simulink model "Target_Control_System"  (R2021b)
settings: Solver=FixedStepDiscrete  StartTime=0.0  StopTime=5  RelTol=1e-3
PreLoadFcn:
  | RTWConfigurationCB('preloadfcn', bdroot);
PostLoadFcn:
  | load('configuration/data_struct.mat');
  | load('configuration/fluxMaps_propMotor.mat');
  | load('configuration/parameterInit_PROP.mat');
  | load('configuration/parameterInit_PUMP.mat');
  | load('configuration/parameterInit_PITCH.mat');
  | load('configuration/parameterInit_TILT.mat');
  | %load('configuration/base_workspace_signal_definition.mat');
  | %load('resolvedatastores_to_baseworkspace_for_faster_simulation.mat');
model workspace (MAT data in the model file):
  SIMULATION_OPTIONS : Simulink.Parameter (value not decoded)
  TARGET_CODE_GEN : Simulink.Parameter (value not decoded)
  TCS_SAMPLE_FREQ_HZ : Simulink.Parameter (value not decoded)
symbols that are objects in the model workspace (value not decoded): TARGET_CODE_GEN, TCS_SAMPLE_FREQ_HZ
undefined symbols (not defined in the file): A_DQ_REF_LPF_INIT__PITCH, A_DQ_REF_LPF_INIT__PROP, A_DQ_REF_LPF_INIT__PUMP, A_DQ_REF_LPF_INIT__TILT, A_OBSERVER_CONFIDENCE_INIT__PITCH, A_OBSERVER_CONFIDENCE_INIT__PROP, A_OBSERVER_CONFIDENCE_INIT__PUMP, A_OBSERVER_CONFIDENCE_INIT__TILT, ACTUATOR_MAX_ANGLE_TRIP__PITCH, ACTUATOR_MIN_ANGLE_TRIP__PITCH, ACTUATOR_POS_SENSOR_INV_DIRECTION__PITCH, ACTUATOR_POS_SENSOR_INV_DIRECTION__TILT, ACTUATOR_POS_SENSOR_OFFSET__PITCH, ACTUATOR_POS_SENSOR_OFFSET__TILT, ADC_scaler1_baseaddr_TILT, ADC_SCALER_FLOAT_TO_FIXPOINT_EXPANSION, ANGLE_ELEC_FROM_SENSOR_OFFSET_INIT__PITCH, ANGLE_ELEC_FROM_SENSOR_OFFSET_INIT__PROP, ANGLE_ELEC_FROM_SENSOR_OFFSET_INIT__PUMP, ANGLE_ELEC_FROM_SENSOR_OFFSET_INIT__TILT, AUTO_CLEAR_FAULTS_ENABLED__PITCH, AUTO_CLEAR_FAULTS_ENABLED__PROP, AUTO_CLEAR_FAULTS_ENABLED__PUMP, AUTO_CLEAR_FAULTS_ENABLED__TILT, AUTO_CLEAR_FAULTS_WAIT_TICKS__PITCH, AUTO_CLEAR_FAULTS_WAIT_TICKS__PROP, AUTO_CLEAR_FAULTS_WAIT_TICKS__PUMP, AUTO_CLEAR_FAULTS_WAIT_TICKS__TILT, AUTO_I_ZERO_IDLE_TICKS__PITCH, AUTO_I_ZERO_IDLE_TICKS__PROP, AUTO_I_ZERO_IDLE_TICKS__PUMP, AUTO_I_ZERO_IDLE_TICKS__TILT, AUTO_I_ZERO_OFFSET_IDC_THRESHOLD__PITCH, AUTO_I_ZERO_OFFSET_IDC_THRESHOLD__PROP, AUTO_I_ZERO_OFFSET_IDC_THRESHOLD__PUMP, AUTO_I_ZERO_OFFSET_IDC_THRESHOLD__TILT, AUTO_I_ZERO_OFFSET_IPH_THRESHOLD__PITCH, AUTO_I_ZERO_OFFSET_IPH_THRESHOLD__PROP, AUTO_I_ZERO_OFFSET_IPH_THRESHOLD__PUMP, AUTO_I_ZERO_OFFSET_IPH_THRESHOLD__TILT, AUTO_SENSORLESS_SWITCHOVER_DISABLE_OMEGA, AUTO_SENSORLESS_SWITCHOVER_ENABLE_OMEGA, AUTO_SENSORLESS_SWITCHOVER_MIN_CONFIDENCE, AUXILIARY_PROTECTION_UNIT_BASEADDR__TILT, blanking_max_error_omega_INIT_PITCH, blanking_max_error_omega_INIT_TILT, blanking_max_error_position_INIT_PITCH, blanking_max_error_position_INIT_TILT, BRUTE_START_I_Q_REF_RAMP_SPEED__PITCH, BRUTE_START_I_Q_REF_RAMP_SPEED__PROP, BRUTE_START_I_Q_REF_RAMP_SPEED__PUMP, BRUTE_START_I_Q_REF_RAMP_SPEED__TILT, CONTROL_LOOP_DT_INIT__PITCH, CONTROL_LOOP_DT_INIT__PROP, CONTROL_LOOP_DT_INIT__PUMP, CONTROL_LOOP_DT_INIT__TILT, CORRECTION_FILTER_SCALE__PITCH, CORRECTION_FILTER_SCALE__PROP, CORRECTION_FILTER_SCALE__PUMP, CORRECTION_FILTER_SCALE__TILT ... (+458)
libraries: simulink x178, Reusables_Lib x24
(part 23 of 47)

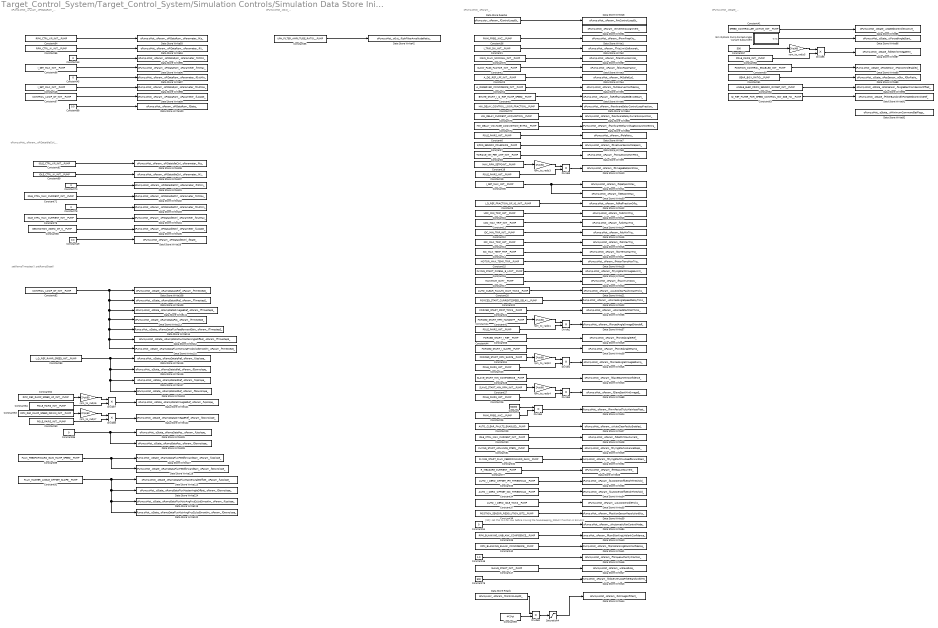
== system Target_Control_System/Target_Control_System/Simulation Controls/Simulation Data Store Initialization/parameter_init_pump/initializeMotorTaskParameterPump() ==
  note: setRampTimestep(); setRampSlope()
  note: oPump.oMot_.oParam_.oPiDataIdleCtrl_...
  note: oPump.oMot_.oParam_.oPiDataRpm_...
  note: oPump.oMot_.oState_...
  note: oPump.oMot_.oParam_...
  note: oPump.oMot_.oOut_...
  note: [SZ]: set this to 0 for now before moving the housekeeping_200Hz() function in Simulink
  Constant : Constant  Value=50000  OutDataTypeStr=single  SampleTime=-1
  Constant1 : Constant  Value=I_TRIP_SW_INIT__PUMP  OutDataTypeStr=single  SampleTime=-1
  Constant10 : Constant  Value=UDC_MIN_TRIP_INIT__PUMP  OutDataTypeStr=single  SampleTime=-1
  Constant11 : Constant  Value=UDC_MAX_TRIP_INIT__PUMP  OutDataTypeStr=single  SampleTime=-1
  Constant12 : Constant  Value=IDC_MIN_TRIP_INIT__PUMP  OutDataTypeStr=single  SampleTime=-1
  Constant13 : Constant  Value=IDC_MAX_TRIP_INIT__PUMP  OutDataTypeStr=single  SampleTime=-1
  Constant14 : Constant  Value=SIC_MAX_TEMP_TRIP__PUMP  OutDataTypeStr=single  SampleTime=-1
  Constant15 : Constant  Value=MOTOR_MAX_TEMP_TRIP__PUMP  OutDataTypeStr=single  SampleTime=-1
  Constant16 : Constant  Value=FLYING_START_OMEGA_E_LIMIT__PUMP  OutDataTypeStr=single  SampleTime=-1
  Constant17 : Constant  Value=MAXIMUM_DUTY__PUMP  OutDataTypeStr=single  SampleTime=-1
  Constant18 : Constant  Value=MAX_RPM_SETPOINT__PUMP  OutDataTypeStr=single  SampleTime=-1
  Constant{6,19,23..24,26,50,58,84} (8 alike) : Constant  Value=POLE_PAIRS_INIT__PUMP  OutDataTypeStr=single  SampleTime=-1
  Constant2 : Constant  Value=SLOW_PASS_FACTOR_INIT__PUMP  OutDataTypeStr=single  SampleTime=-1
  Constant20 : Constant  Value=AUTO_CLEAR_FAULTS_WAIT_TICKS__PUMP  OutDataTypeStr=uint32  SampleTime=-1
  Constant21 : Constant  Value=FORCED_START_POST_TICKS__PUMP  OutDataTypeStr=uint32  SampleTime=-1
  Constant22 : Constant  Value=FORCED_START_CURRENT2SPEED_DELAY__PUMP  OutDataTypeStr=uint32  SampleTime=-1
  Constant25 : Constant  Value=PWM_FREQ_KHZ__PUMP  OutDataTypeStr=single  SampleTime=-1
  Constant27 : Constant  Value=SLAVE_START_MIN_RPM_INIT__PUMP  OutDataTypeStr=single  SampleTime=-1
  Constant28 : Constant  Value=SLAVE_START_MIN_CONFIDENCE__PUMP  OutDataTypeStr=single  SampleTime=-1
  Constant29 : Constant  Value=AUTO_CLEAR_FAULTS_ENABLED__PUMP  OutDataTypeStr=uint32  SampleTime=-1
  Constant3 : Constant  Value=A_DQ_REF_LPF_INIT__PUMP  OutDataTypeStr=single  SampleTime=-1
  Constant30 : Constant  Value=IDLE_CTRL_MAX_CURRENT_INIT__PUMP  OutDataTypeStr=single  SampleTime=-1
  Constant31 : Constant  Value=FLYING_START_ADVANCE_STEPS__PUMP  OutDataTypeStr=single  SampleTime=-1
  Constant32 : Constant  Value=FLYING_START_FLUX_FEEDFORWARD_GAIN__PUMP  OutDataTypeStr=single  SampleTime=-1
  Constant33 : Constant  Value=AUTO_I_ZERO_OFFSET_IPH_THRESHOLD__PUMP  OutDataTypeStr=single  SampleTime=-1
  Constant34 : Constant  Value=AUTO_I_ZERO_OFFSET_IDC_THRESHOLD__PUMP  VectorParams1D=off  OutDataTypeStr=single  SampleTime=-1
  Constant35 : Constant  Value=I_SET_MAX_INIT__PUMP  OutDataTypeStr=single  SampleTime=-1
  Constant36 : Constant  Value=PWM_FREQ_KHZ__PUMP  OutDataTypeStr=single  SampleTime=-1
  Constant37 : Constant  Value=AUTO_I_ZERO_IDLE_TICKS__PUMP  OutDataTypeStr=uint32  SampleTime=-1
  Constant38 : Constant  Value=POSITION_SENSOR_RESOLUTION_BITS__PUMP  OutDataTypeStr=single  SampleTime=-1
  Constant39 : Constant  Value=RPM_BLANKING_UNBLANK_CONFIDENCE__PUMP  OutDataTypeStr=single  SampleTime=-1
  Constant4 : Constant  Value=A_OBSERVER_CONFIDENCE_INIT__PUMP  OutDataTypeStr=single  SampleTime=-1
  Constant40 : Constant  Value=RPM_BLANKING_BLANK_CONFIDENCE__PUMP  OutDataTypeStr=single  SampleTime=-1
  Constant41 : Constant  Value=SPEED_CONTROLLER_ACTIVE_INIT__PUMP  OutDataTypeStr=uint32  SampleTime=-1
  Constant42 : Constant  Value=FORCED_START_RPM_HANDOFF__PUMP  OutDataTypeStr=single  SampleTime=-1
  Constant{43,45,70,78,86} (5 alike) : Constant  Value=0  OutDataTypeStr=single  SampleTime=-1
  Constant44 : Constant  Value=FORCED_START_I_SLOPE__PUMP  OutDataTypeStr=single  SampleTime=-1
  Constant46 : Constant  Value=1.0  OutDataTypeStr=single  SampleTime=-1
  Constant47 : Constant  Value=SLAVE_START_INIT__PUMP  OutDataTypeStr=uint32  SampleTime=-1
  Constant48 : Constant  Value=I_SET_MAX_INIT__PUMP  OutDataTypeStr=single  SampleTime=-1
  Constant49 : Constant  Value=0.0  OutDataTypeStr=single  SampleTime=-1
  Constant5 : Constant  Value=BRUTE_START_I_Q_REF_RAMP_SPEED__PUMP  OutDataTypeStr=single  SampleTime=-1
  Constant51 : Constant  Value=FORCED_START_RPM_SLOPE__PUMP  OutDataTypeStr=single  SampleTime=-1
  Constant52 : Constant  Value=RPM_REF_RAMP_SPEED_UP_INIT__PUMP  OutDataTypeStr=single  SampleTime=-1
  Constant53 : Constant  Value=RPM_REF_RAMP_SPEED_DOWN_INIT__PUMP  OutDataTypeStr=single  SampleTime=-1
  Constant54 : Constant  Value=0  OutDataTypeStr=uint32  SampleTime=-1
  Constant55 : Constant  Value=UPH_FILTER_AMPLITUDE_RATIO__PUMP  VectorParams1D=off  OutDataTypeStr=single  SampleTime=-1
  Constant56 : Constant  Value=FORCED_START_I_REF__PUMP  OutDataTypeStr=single  SampleTime=-1
  Constant57 : Constant  Value=500  OutDataTypeStr=single  SampleTime=-1
  Constant59 : Constant  Value=4*2*pi  OutDataTypeStr=single  SampleTime=-1
  Constant60 : Constant  Value=POSITION_CONTROL_ENABLED_INIT__PUMP  OutDataTypeStr=int32  SampleTime=-1
  Constant61 : Constant  Value=GEAR_BOX_RATIO__PUMP  OutDataTypeStr=single  SampleTime=-1
  Constant62 : Constant  Value=ANGLE_ELEC_FROM_SENSOR_OFFSET_INIT__PUMP  OutDataTypeStr=single  SampleTime=-1
  Constant63 : Constant  Value=IQ_REF_FILTER_FOR_SPEED_CONTROL_BW_3DB_HZ__PUMP  OutDataTypeStr=single  SampleTime=-1
  Constant64 : Constant  Value=RPM_CTRL_KP_INIT__PUMP  OutDataTypeStr=single  SampleTime=-1
  Constant65 : Constant  Value=RPM_CTRL_KI_INIT__PUMP  OutDataTypeStr=single  SampleTime=-1
  Constant66 : Constant  Value=I_SET_MAX_INIT__PUMP  OutDataTypeStr=single  SampleTime=-1
  Constant67 : Constant  Value=CONTROL_LOOP_DT_INIT__PUMP  OutDataTypeStr=single  SampleTime=-1
  Constant68 : Constant  Value=0.0  OutDataTypeStr=single  SampleTime=-1
  Constant69 : Constant  Value=IDLE_CTRL_KI_INIT__PUMP  OutDataTypeStr=single  SampleTime=-1
  Constant7 : Constant  Value=1/POS_SENSOR_POLEPAIRS__PUMP  OutDataTypeStr=single  SampleTime=-1
  Constant71 : Constant  Value=IDLE_CTRL_MAX_CURRENT_INIT__PUMP  OutDataTypeStr=single  SampleTime=-1
  Constant72 : Constant  Value=HW_DELAY_CONTROL_LOOP_FRACTION__PUMP  OutDataTypeStr=single  SampleTime=-1
  Constant73 : Constant  Value=HW_DELAY_CURRENT_ACQUISITION__PUMP  OutDataTypeStr=single  SampleTime=-1
  Constant74 : Constant  Value=HW_DELAY_VOLTAGE_ACQUISITION_EXTRA__PUMP  OutDataTypeStr=single  SampleTime=-1
  Constant75 : Constant  Value=MAIN_FLUX_NOMINAL_INIT__PUMP  OutDataTypeStr=single  SampleTime=-1
  Constant76 : Constant  Value=500  OutDataTypeStr=single  SampleTime=-1
  Constant77 : Constant  Value=R_MEASURE_CURRENT__PUMP  OutDataTypeStr=single  SampleTime=-1
  Constant79 : Constant  Value=IDLE_CTRL_MAX_CURRENT_INIT__PUMP  VectorParams1D=off  OutDataTypeStr=single  SampleTime=-1
  Constant8 : Constant  Value=TORQUE_NM_PER_AMP_INIT__PUMP  OutDataTypeStr=single  SampleTime=-1
  Constant80 : Constant  Value=DECIMATION_200HZ_DT_S__PUMP  OutDataTypeStr=single  SampleTime=-1
  Constant81 : Constant  Value=IDLE_CTRL_KP_INIT__PUMP  OutDataTypeStr=single  SampleTime=-1
  Constant82 : Constant  Value=CONTROL_LOOP_DT_INIT__PUMP  OutDataTypeStr=single  SampleTime=-1
  Constant83 : Constant  Value=I_Q_REF_RAMP_SPEED_INIT__PUMP  OutDataTypeStr=single  SampleTime=-1
  Constant89 : Constant  Value=FLUX_FEEDFORWARD_GAIN_RAMP_SPEED__PUMP  OutDataTypeStr=single  SampleTime=-1
  Constant9 : Constant  Value=I_D_REF_FRACTION_OF_IQ_INIT__PUMP  OutDataTypeStr=single  SampleTime=-1
  Constant92 : Constant  Value=FLUX_MASTER_ANGLE_OFFSET_SLOPE__PUMP  OutDataTypeStr=single  SampleTime=-1
  Data Store Read1 : DataStoreRead  DataStoreName=oPump  DataStoreElements=oPump.oIsr_.oParam_.fControlLoopDt_  IndexOptions=Index vector (dialog)  Indices=1  OutputSizes=1
  Data Store Read14 : DataStoreRead  DataStoreName=oPump  DataStoreElements=oPump.oIsr_.oParam_.fControlLoopDt_  IndexOptions=Index vector (dialog)  Indices=1  OutputSizes=1
  Data Store Write1 : DataStoreWrite  DataStoreName=oPump  DataStoreElements=oPump.oMot_.oParam_.fPwmFreqKhz_  IndexOptions=Index vector (dialog)  Indices=1  OutputSizes=1
  Data Store Write10 : DataStoreWrite  DataStoreName=oPump  DataStoreElements=oPump.oMot_.oParam_.fOmegaESetpointMax_  IndexOptions=Index vector (dialog)  Indices=1  OutputSizes=1
  Data Store Write100 : DataStoreWrite  DataStoreName=oPump  DataStoreElements=oPump.oMot_.oParam_.oPiDataRpm_.fState_  IndexOptions=Index vector (dialog)  Indices=1  OutputSizes=1
  Data Store Write101 : DataStoreWrite  DataStoreName=oPump  DataStoreElements=oPump.oMot_.oParam_.oPiDataIdleCtrl_.oParameter_.fIntMin_  IndexOptions=Index vector (dialog)  Indices=1  OutputSizes=1
  Data Store Write102 : DataStoreWrite  DataStoreName=oPump  DataStoreElements=oPump.oMot_.oParam_.oPiDataIdleCtrl_.oParameter_.fIntMax_  IndexOptions=Index vector (dialog)  Indices=1  OutputSizes=1
  Data Store Write103 : DataStoreWrite  DataStoreName=oPump  DataStoreElements=oPump.oMot_.oParam_.oPiDataIdleCtrl_.oParameter_.fOutMin_  IndexOptions=Index vector (dialog)  Indices=1  OutputSizes=1
  Data Store Write104 : DataStoreWrite  DataStoreName=oPump  DataStoreElements=oPump.oMot_.oParam_.oPiDataIdleCtrl_.oParameter_.fOutMax_  IndexOptions=Index vector (dialog)  Indices=1  OutputSizes=1
  Data Store Write105 : DataStoreWrite  DataStoreName=oPump  DataStoreElements=oPump.oMot_.oParam_.oPiDataIdleCtrl_.oParameter_.fLoopDt_  IndexOptions=Index vector (dialog)  Indices=1  OutputSizes=1
  Data Store Write106 : DataStoreWrite  DataStoreName=oPump  DataStoreElements=oPump.oMot_.oParam_.oPiDataIdleCtrl_.oParameter_.fKp_  IndexOptions=Index vector (dialog)  Indices=1  OutputSizes=1
  Data Store Write107 : DataStoreWrite  DataStoreName=oPump  DataStoreElements=oPump.oMot_.oParam_.oPiDataIdleCtrl_.oParameter_.fKi_  IndexOptions=Index vector (dialog)  Indices=1  OutputSizes=1
  Data Store Write108 : DataStoreWrite  DataStoreName=oPump  DataStoreElements=oPump.oMot_.oState_.oRampDataIqRef_.oParam_.fTimestepS_  IndexOptions=Index vector (dialog)  Indices=1  OutputSizes=1
  Data Store Write109 : DataStoreWrite  DataStoreName=oPump  DataStoreElements=oPump.oMot_.oState_.oRampDataIdRef_.oParam_.fTimestepS_  IndexOptions=Index vector (dialog)  Indices=1  OutputSizes=1
  Data Store Write11 : DataStoreWrite  DataStoreName=oPump  DataStoreElements=oPump.oMot_.oParam_.fIqSetpointMax_  IndexOptions=Index vector (dialog)  Indices=1  OutputSizes=1
  Data Store Write110 : DataStoreWrite  DataStoreName=oPump  DataStoreElements=oPump.oMot_.oState_.oRampDataFluxMstrAngFrcd2clsdSmoothn_.oParam_.fTimestepS_  IndexOptions=Index vector (dialog)  Indices=1  OutputSizes=1
  Data Store Write111 : DataStoreWrite  DataStoreName=oPump  DataStoreElements=oPump.oMot_.oState_.oRampDataOmegaERef_.oParam_.fTimestepS_  IndexOptions=Index vector (dialog)  Indices=1  OutputSizes=1
  Data Store Write112 : DataStoreWrite  DataStoreName=oPump  DataStoreElements=oPump.oMot_.oState_.oRampDataFluxMasterAngleOffset_.oParam_.fTimestepS_  IndexOptions=Index vector (dialog)  Indices=1  OutputSizes=1
  Data Store Write113 : DataStoreWrite  DataStoreName=oPump  DataStoreElements=oPump.oMot_.oState_.oRampDataPos_.oParam_.fTimestepS_  IndexOptions=Index vector (dialog)  Indices=1  OutputSizes=1
  Data Store Write114 : DataStoreWrite  DataStoreName=oPump  DataStoreElements=oPump.oMot_.oState_.oRampDataFluxFeedforwardGain_.oParam_.fTimestepS_  IndexOptions=Index vector (dialog)  Indices=1  OutputSizes=1
  Data Store Write115 : DataStoreWrite  DataStoreName=oPump  DataStoreElements=oPump.oMot_.oState_.oRampDataIqRef_.oParam_.fUpslope_  IndexOptions=Index vector (dialog)  Indices=1  OutputSizes=1
  Data Store Write116 : DataStoreWrite  DataStoreName=oPump  DataStoreElements=oPump.oMot_.oState_.oRampDataIqRef_.oParam_.fDownslope_  IndexOptions=Index vector (dialog)  Indices=1  OutputSizes=1
  Data Store Write117 : DataStoreWrite  DataStoreName=oPump  DataStoreElements=oPump.oMot_.oState_.oRampDataIdRef_.oParam_.fUpslope_  IndexOptions=Index vector (dialog)  Indices=1  OutputSizes=1
  Data Store Write118 : DataStoreWrite  DataStoreName=oPump  DataStoreElements=oPump.oMot_.oState_.oRampDataIdRef_.oParam_.fDownslope_  IndexOptions=Index vector (dialog)  Indices=1  OutputSizes=1
  Data Store Write119 : DataStoreWrite  DataStoreName=oPump  DataStoreElements=oPump.oMot_.oState_.oRampDataFluxMstrAngFrcd2clsdSmoothn_.oParam_.fUpslope_  IndexOptions=Index vector (dialog)  Indices=1  OutputSizes=1
  Data Store Write12 : DataStoreWrite  DataStoreName=oPump  DataStoreElements=oPump.oMot_.oParam_.fIdRefFractionOfIq_  IndexOptions=Index vector (dialog)  Indices=1  OutputSizes=1
  Data Store Write120 : DataStoreWrite  DataStoreName=oPump  DataStoreElements=oPump.oMot_.oState_.oRampDataFluxMstrAngFrcd2clsdSmoothn_.oParam_.fDownslope_  IndexOptions=Index vector (dialog)  Indices=1  OutputSizes=1
  Data Store Write121 : DataStoreWrite  DataStoreName=oPump  DataStoreElements=oPump.oMot_.oState_.oRampDataOmegaERef_.oParam_.fUpslope_  IndexOptions=Index vector (dialog)  Indices=1  OutputSizes=1
  Data Store Write122 : DataStoreWrite  DataStoreName=oPump  DataStoreElements=oPump.oMot_.oState_.oRampDataOmegaERef_.oParam_.fDownslope_  IndexOptions=Index vector (dialog)  Indices=1  OutputSizes=1
  Data Store Write123 : DataStoreWrite  DataStoreName=oPump  DataStoreElements=oPump.oMot_.oState_.oRampDataFluxMasterAngleOffset_.oParam_.fUpslope_  IndexOptions=Index vector (dialog)  Indices=1  OutputSizes=1
  Data Store Write124 : DataStoreWrite  DataStoreName=oPump  DataStoreElements=oPump.oMot_.oState_.oRampDataFluxMasterAngleOffset_.oParam_.fDownslope_  IndexOptions=Index vector (dialog)  Indices=1  OutputSizes=1
  Data Store Write125 : DataStoreWrite  DataStoreName=oPump  DataStoreElements=oPump.oMot_.oState_.oRampDataPos_.oParam_.fUpslope_  IndexOptions=Index vector (dialog)  Indices=1  OutputSizes=1
  Data Store Write126 : DataStoreWrite  DataStoreName=oPump  DataStoreElements=oPump.oMot_.oState_.oRampDataPos_.oParam_.fDownslope_  IndexOptions=Index vector (dialog)  Indices=1  OutputSizes=1
  Data Store Write127 : DataStoreWrite  DataStoreName=oPump  DataStoreElements=oPump.oMot_.oState_.oRampDataFluxFeedforwardGain_.oParam_.fUpslope_  IndexOptions=Index vector (dialog)  Indices=1  OutputSizes=1
  Data Store Write128 : DataStoreWrite  DataStoreName=oPump  DataStoreElements=oPump.oMot_.oState_.oRampDataFluxFeedforwardGain_.oParam_.fDownslope_  IndexOptions=Index vector (dialog)  Indices=1  OutputSizes=1
  Data Store Write13 : DataStoreWrite  DataStoreName=oPump  DataStoreElements=oPump.oMot_.oParam_.fUdcMinTrip_  IndexOptions=Index vector (dialog)  Indices=1  OutputSizes=1
  Data Store Write14 : DataStoreWrite  DataStoreName=oPump  DataStoreElements=oPump.oMot_.oParam_.fUdcMaxTrip_  IndexOptions=Index vector (dialog)  Indices=1  OutputSizes=1
  Data Store Write15 : DataStoreWrite  DataStoreName=oPump  DataStoreElements=oPump.oMot_.oParam_.fIdcMinTrip_  IndexOptions=Index vector (dialog)  Indices=1  OutputSizes=1
  Data Store Write16 : DataStoreWrite  DataStoreName=oPump  DataStoreElements=oPump.oMot_.oParam_.fIdcMaxTrip_  IndexOptions=Index vector (dialog)  Indices=1  OutputSizes=1
  Data Store Write17 : DataStoreWrite  DataStoreName=oPump  DataStoreElements=oPump.oMot_.oParam_.fSicTempMaxTrip_  IndexOptions=Index vector (dialog)  Indices=1  OutputSizes=1
  Data Store Write18 : DataStoreWrite  DataStoreName=oPump  DataStoreElements=oPump.oMot_.oParam_.fMotorTempMaxTrip_  IndexOptions=Index vector (dialog)  Indices=1  OutputSizes=1
  Data Store Write19 : DataStoreWrite  DataStoreName=oPump  DataStoreElements=oPump.oMot_.oParam_.fFlyingStartOmegaELimit_  IndexOptions=Index vector (dialog)  Indices=1  OutputSizes=1
  Data Store Write2 : DataStoreWrite  DataStoreName=oPump  DataStoreElements=oPump.oMot_.oParam_.fTripLimitSoftwareA_  IndexOptions=Index vector (dialog)  Indices=1  OutputSizes=1
  Data Store Write20 : DataStoreWrite  DataStoreName=oPump  DataStoreElements=oPump.oMot_.oParam_.fMaximumDuty_  IndexOptions=Index vector (dialog)  Indices=1  OutputSizes=1
  Data Store Write21 : DataStoreWrite  DataStoreName=oPump  DataStoreElements=oPump.oMot_.oParam_.uiAutoClearFaultsWaitTicks_  IndexOptions=Index vector (dialog)  Indices=1  OutputSizes=1
  Data Store Write22 : DataStoreWrite  DataStoreName=oPump  DataStoreElements=oPump.oMot_.oParam_.uiForcedAngleSpeedDelayTicks_  IndexOptions=Index vector (dialog)  Indices=1  OutputSizes=1
  Data Store Write23 : DataStoreWrite  DataStoreName=oPump  DataStoreElements=oPump.oMot_.oParam_.fSlaveStartMinConfidence_  IndexOptions=Index vector (dialog)  Indices=1  OutputSizes=1
  Data Store Write24 : DataStoreWrite  DataStoreName=oPump  DataStoreElements=oPump.oMot_.oParam_.fPwmPeriodTicksMainloopFloat_  IndexOptions=Index vector (dialog)  Indices=1  OutputSizes=1
  Data Store Write25 : DataStoreWrite  DataStoreName=oPump  DataStoreElements=oPump.oMot_.oParam_.fRMeasureCurrent_  IndexOptions=Index vector (dialog)  Indices=1  OutputSizes=1
  Data Store Write26 : DataStoreWrite  DataStoreName=oPump  DataStoreElements=oPump.oMot_.oParam_.oPiDataIdleCtrl_.fState_  IndexOptions=Index vector (dialog)  Indices=1  OutputSizes=1
  Data Store Write27 : DataStoreWrite  DataStoreName=oPump  DataStoreElements=oPump.oMot_.oParam_.uiAutoClearFaultsEnabled_  IndexOptions=Index vector (dialog)  Indices=1  OutputSizes=1
  Data Store Write28 : DataStoreWrite  DataStoreName=oPump  DataStoreElements=oPump.oMot_.oParam_.fIdleCtrlMaxCurrent_  IndexOptions=Index vector (dialog)  Indices=1  OutputSizes=1
  Data Store Write29 : DataStoreWrite  DataStoreName=oPump  DataStoreElements=oPump.oMot_.oParam_.fFlyingStartAdvanceSteps_  IndexOptions=Index vector (dialog)  Indices=1  OutputSizes=1
  Data Store Write3 : DataStoreWrite  DataStoreName=oPump  DataStoreElements=oPump.oMot_.oParam_.fSlowPassFactor_  IndexOptions=Index vector (dialog)  Indices=1  OutputSizes=1
  Data Store Write30 : DataStoreWrite  DataStoreName=oPump  DataStoreElements=oPump.oMot_.oParam_.fISetpointMax_  IndexOptions=Index vector (dialog)  Indices=1  OutputSizes=1
  Data Store Write31 : DataStoreWrite  DataStoreName=oPump  DataStoreElements=oPump.oMot_.oParam_.eInverterAssignment_  IndexOptions=Index vector (dialog)  Indices=1  OutputSizes=1
  Data Store Write32 : DataStoreWrite  DataStoreName=oPump  DataStoreElements=oPump.oMot_.oParam_.fFlyingStartFluxFeedforwardGain_  IndexOptions=Index vector (dialog)  Indices=1  OutputSizes=1
  Data Store Write33 : DataStoreWrite  DataStoreName=oPump  DataStoreElements=oPump.oMot_.oParam_.fAutoIZeroOffsetIphThreshold_  IndexOptions=Index vector (dialog)  Indices=1  OutputSizes=1
  Data Store Write34 : DataStoreWrite  DataStoreName=oPump  DataStoreElements=oPump.oMot_.oParam_.fAutoIZeroOffsetIdcThreshold_  IndexOptions=Index vector (dialog)  Indices=1  OutputSizes=1
  Data Store Write35 : DataStoreWrite  DataStoreName=oPump  DataStoreElements=oPump.oMot_.oParam_.uiAutoIZeroIdleTicks_  IndexOptions=Index vector (dialog)  Indices=1  OutputSizes=1
  Data Store Write36 : DataStoreWrite  DataStoreName=oPump  DataStoreElements=oPump.oMot_.oParam_.uiForcedStartPostTicks_  IndexOptions=Index vector (dialog)  Indices=1  OutputSizes=1
  Data Store Write37 : DataStoreWrite  DataStoreName=oPump  DataStoreElements=oPump.oMot_.oParam_.fForcedAngleOmegaEHandoff_  IndexOptions=Index vector (dialog)  Indices=1  OutputSizes=1
  Data Store Write38 : DataStoreWrite  DataStoreName=oPump  DataStoreElements=oPump.oMot_.oParam_.fForcedAngleIRamp_  IndexOptions=Index vector (dialog)  Indices=1  OutputSizes=1
  Data Store Write39 : DataStoreWrite  DataStoreName=oPump  DataStoreElements=oPump.oMot_.oParam_.fPositionSensorResolutionBits_  IndexOptions=Index vector (dialog)  Indices=1  OutputSizes=1
  Data Store Write4 : DataStoreWrite  DataStoreName=oPump  DataStoreElements=oPump.oMot_.oParam_.fADqRefLpf_  IndexOptions=Index vector (dialog)  Indices=1  OutputSizes=1
  Data Store Write40 : DataStoreWrite  DataStoreName=oPump  DataStoreElements=oPump.oMot_.oParam_.fRpmBlankingUnblankConfidence_  IndexOptions=Index vector (dialog)  Indices=1  OutputSizes=1
  Data Store Write41 : DataStoreWrite  DataStoreName=oPump  DataStoreElements=oPump.oMot_.oParam_.fRpmBlankingBlankConfidence_  IndexOptions=Index vector (dialog)  Indices=1  OutputSizes=1
  Data Store Write42 : DataStoreWrite  DataStoreName=oPump  DataStoreElements=oPump.oMot_.oOut_.fUphFilterAmplitudeRatio_  IndexOptions=Index vector (dialog)  Indices=1  OutputSizes=1
  Data Store Write43 : DataStoreWrite  DataStoreName=oPump  DataStoreElements=oPump.oMot_.oParam_.fObserverLoopFilterBandwidthHz_  IndexOptions=Index vector (dialog)  Indices=1  OutputSizes=1
  Data Store Write44 : DataStoreWrite  DataStoreName=oPump  DataStoreElements=oPump.oMot_.oParam_.fAOmegaXfilter2_  IndexOptions=Index vector (dialog)  Indices=1  OutputSizes=1
  Data Store Write45 : DataStoreWrite  DataStoreName=oPump  DataStoreElements=oPump.oMot_.oParam_.fForcedAngleOmegaERamp_  IndexOptions=Index vector (dialog)  Indices=1  OutputSizes=1
  Data Store Write46 : DataStoreWrite  DataStoreName=oPump  DataStoreElements=oPump.oMot_.oParam_.fTorqueAuthorityFraction_  IndexOptions=Index vector (dialog)  Indices=1  OutputSizes=1
  Data Store Write47 : DataStoreWrite  DataStoreName=oPump  DataStoreElements=oPump.oMot_.oParam_.uiSlaveRole_  IndexOptions=Index vector (dialog)  Indices=1  OutputSizes=1
  Data Store Write48 : DataStoreWrite  DataStoreName=oPump  DataStoreElements=oPump.oMot_.oParam_.fIntControlLoopDt_  IndexOptions=Index vector (dialog)  Indices=1  OutputSizes=1
  Data Store Write49 : DataStoreWrite  DataStoreName=oPump  DataStoreElements=oPump.oMot_.oParam_.fForcedAngleIRef_  IndexOptions=Index vector (dialog)  Indices=1  OutputSizes=1
  Data Store Write5 : DataStoreWrite  DataStoreName=oPump  DataStoreElements=oPump.oMot_.oParam_.fAObserverConfidence_  IndexOptions=Index vector (dialog)  Indices=1  OutputSizes=1
  Data Store Write6 : DataStoreWrite  DataStoreName=oPump  DataStoreElements=oPump.oMot_.oParam_.fIqRefRampSpeedBruteStart_  IndexOptions=Index vector (dialog)  Indices=1  OutputSizes=1
  Data Store Write64 : DataStoreWrite  DataStoreName=oPump  DataStoreElements=oPump.oMot_.oParam_.fHardwareDelayControlLoopFraction_  IndexOptions=Index vector (dialog)  Indices=1  OutputSizes=1
  Data Store Write65 : DataStoreWrite  DataStoreName=oPump  DataStoreElements=oPump.oMot_.oParam_.fHardwareDelayCurrentAcquisition_  IndexOptions=Index vector (dialog)  Indices=1  OutputSizes=1
  Data Store Write66 : DataStoreWrite  DataStoreName=oPump  DataStoreElements=oPump.oMot_.oParam_.fHardwareDelayVoltageAcquisitionExtra_  IndexOptions=Index vector (dialog)  Indices=1  OutputSizes=1
  Data Store Write67 : DataStoreWrite  DataStoreName=oPump  DataStoreElements=oPump.oMot_.oParam_.fMainFluxNominal_  IndexOptions=Index vector (dialog)  Indices=1  OutputSizes=1
  Data Store Write69 : DataStoreWrite  DataStoreName=oPump  DataStoreElements=oPump.oMot_.oParam_.fSlaveStartMinOmegaE_  IndexOptions=Index vector (dialog)  Indices=1  OutputSizes=1
  Data Store Write7 : DataStoreWrite  DataStoreName=oPump  DataStoreElements=oPump.oMot_.oParam_.fPolePairs_  IndexOptions=Index vector (dialog)  Indices=1  OutputSizes=1
  Data Store Write8 : DataStoreWrite  DataStoreName=oPump  DataStoreElements=oPump.oMot_.oParam_.fOneOverSensorPolepairs_  IndexOptions=Index vector (dialog)  Indices=1  OutputSizes=1
  Data Store Write84 : DataStoreWrite  DataStoreName=oPump  DataStoreElements=oPump.oMot_.oParam_.uiAutomaticFanControlMode_  IndexOptions=Index vector (dialog)  Indices=1  OutputSizes=1
  Data Store Write85 : DataStoreWrite  DataStoreName=oPump  DataStoreElements=oPump.oMot_.oState_.uiSpeedControllerActive_  IndexOptions=Index vector (dialog)  Indices=1  OutputSizes=1
  Data Store Write86 : DataStoreWrite  DataStoreName=oPump  DataStoreElements=oPump.oMot_.oState_.uiForcedAngleStart_  IndexOptions=Index vector (dialog)  Indices=1  OutputSizes=1
  Data Store Write87 : DataStoreWrite  DataStoreName=oPump  DataStoreElements=oPump.oMot_.oState_.fIdleCtrlOmegaEMin_  IndexOptions=Index vector (dialog)  Indices=1  OutputSizes=1
  Data Store Write88 : DataStoreWrite  DataStoreName=oPump  DataStoreElements=oPump.oMot_.oState_.oPosSensor_.iPosControlEnabled_  IndexOptions=Index vector (dialog)  Indices=1  OutputSizes=1
  Data Store Write89 : DataStoreWrite  DataStoreName=oPump  DataStoreElements=oPump.oMot_.oState_.oPosSensor_.oGbx_.fGbxRatio_  IndexOptions=Index vector (dialog)  Indices=1  OutputSizes=1
  Data Store Write9 : DataStoreWrite  DataStoreName=oPump  DataStoreElements=oPump.oMot_.oParam_.fTorqueConstNmPerA_  IndexOptions=Index vector (dialog)  Indices=1  OutputSizes=1
  Data Store Write90 : DataStoreWrite  DataStoreName=oPump  DataStoreElements=oPump.oMot_.oState_.oPosSensor_.fAngleElecFromSensorOffset_  IndexOptions=Index vector (dialog)  Indices=1  OutputSizes=1
  Data Store Write91 : DataStoreWrite  DataStoreName=oPump  DataStoreElements=oPump.oMot_.oState_.fFilterBandwidthForSpeedControlIqRef_  IndexOptions=Index vector (dialog)  Indices=1  OutputSizes=1
  Data Store Write92 : DataStoreWrite  DataStoreName=oPump  DataStoreElements=oPump.oMot_.oState_.uiMinimumCommandSetFlags_  IndexOptions=Index vector (dialog)  Indices=1  OutputSizes=1
  Data Store Write93 : DataStoreWrite  DataStoreName=oPump  DataStoreElements=oPump.oMot_.oParam_.oPiDataRpm_.oParameter_.fKp_  IndexOptions=Index vector (dialog)  Indices=1  OutputSizes=1
  Data Store Write94 : DataStoreWrite  DataStoreName=oPump  DataStoreElements=oPump.oMot_.oParam_.oPiDataRpm_.oParameter_.fKi_  IndexOptions=Index vector (dialog)  Indices=1  OutputSizes=1
  Data Store Write95 : DataStoreWrite  DataStoreName=oPump  DataStoreElements=oPump.oMot_.oParam_.oPiDataRpm_.oParameter_.fIntMin_  IndexOptions=Index vector (dialog)  Indices=1  OutputSizes=1
  Data Store Write96 : DataStoreWrite  DataStoreName=oPump  DataStoreElements=oPump.oMot_.oParam_.oPiDataRpm_.oParameter_.fIntMax_  IndexOptions=Index vector (dialog)  Indices=1  OutputSizes=1
  Data Store Write97 : DataStoreWrite  DataStoreName=oPump  DataStoreElements=oPump.oMot_.oParam_.oPiDataRpm_.oParameter_.fOutMin_  IndexOptions=Index vector (dialog)  Indices=1  OutputSizes=1
  Data Store Write98 : DataStoreWrite  DataStoreName=oPump  DataStoreElements=oPump.oMot_.oParam_.oPiDataRpm_.oParameter_.fOutMax_  IndexOptions=Index vector (dialog)  Indices=1  OutputSizes=1
  Data Store Write99 : DataStoreWrite  DataStoreName=oPump  DataStoreElements=oPump.oMot_.oParam_.oPiDataRpm_.oParameter_.fLoopDt_  IndexOptions=Index vector (dialog)  Indices=1  OutputSizes=1
  Divide{1..8} (8 alike) : Product  Inputs=**  OutDataTypeStr=single
  Divide9 : Product  Inputs=**
  Saturation4 : Saturate  UpperLimit=1.0  LowerLimit=1e-6
  Sim Options Pump Forced Angle Variant Subsystem : Subsystem  Variant=on
  rpm_to_rad/s{1..7} (7 alike) : Gain  Gain=2*pi/60  OutDataTypeStr=single
  wires:
  Saturation4/1 -> Data Store Write44/1
  Divide9/1 -> Saturation4/1
  Constant59/1 -> Divide9/2
  Data Store Read1/1 -> Divide9/1
  Data Store Read14/1 -> Data Store Write48/1
  Constant76/1 -> Data Store Write43/1
  Constant55/1 -> Data Store Write42/1
  Constant53/1 -> rpm_to_rad/s7/1
  Constant52/1 -> rpm_to_rad/s6/1
  Divide8/1 -> Data Store Write122/1
  rpm_to_rad/s7/1 -> Divide8/1
  Constant50/1 -> Divide8/2
  Constant49/1 -> Data Store Write26/1
  Constant48/1 -> Data Store Write98/1
  Constant45/1 -> Data Store Write97/1
  Constant43/1 -> Data Store Write95/1
  Constant79/1 -> Data Store Write104/1
  Constant92/1 -> Data Store Write123/1, Data Store Write120/1, Data Store Write119/1, Data Store Write124/1
  Constant64/1 -> Data Store Write93/1
  Constant80/1 -> Data Store Write105/1
  Constant89/1 -> Data Store Write127/1, Data Store Write128/1
  Constant86/1 -> Data Store Write125/1, Data Store Write126/1
  Constant69/1 -> Data Store Write107/1
  Constant81/1 -> Data Store Write106/1
  Constant83/1 -> Data Store Write115/1, Data Store Write118/1, Data Store Write117/1, Data Store Write116/1
  Constant70/1 -> Data Store Write101/1
  rpm_to_rad/s6/1 -> Divide7/1
  Constant71/1 -> Data Store Write102/1
  Constant67/1 -> Data Store Write99/1
  Constant84/1 -> Divide7/2
  Constant78/1 -> Data Store Write103/1
  Constant66/1 -> Data Store Write96/1
  Divide7/1 -> Data Store Write121/1
  Constant68/1 -> Data Store Write100/1
  Constant65/1 -> Data Store Write94/1
  Constant82/1 -> Data Store Write110/1, Data Store Write112/1, Data Store Write114/1, Data Store Write113/1, Data Store Write111/1, Data Store Write109/1, Data Store Write108/1
  Constant57/1 -> rpm_to_rad/s5/1
  rpm_to_rad/s5/1 -> Divide6/1
  Constant63/1 -> Data Store Write91/1
  Constant41/1 -> Data Store Write85/1
  Constant61/1 -> Data Store Write89/1
  Constant58/1 -> Divide6/2
  Constant60/1 -> Data Store Write88/1
  Sim Options Pump Forced Angle Variant Subsystem/1(Out1) -> Data Store Write86/1
  Divide6/1 -> Data Store Write87/1
  Constant62/1 -> Data Store Write90/1
  Constant54/1 -> Data Store Write84/1
  Constant46/1 -> Data Store Write46/1
  Constant13/1 -> Data Store Write16/1
  Constant5/1 -> Data Store Write6/1
  Constant24/1 -> Divide2/2
  Constant33/1 -> Data Store Write33/1
  Constant31/1 -> Data Store Write29/1
  Constant16/1 -> Data Store Write19/1
  Constant18/1 -> rpm_to_rad/s3/1
  Constant37/1 -> Data Store Write35/1
  Constant40/1 -> Data Store Write41/1
  Divide5/1 -> Data Store Write69/1
  rpm_to_rad/s3/1 -> Divide3/1
  Constant47/1 -> Data Store Write47/1
  Constant2/1 -> Data Store Write3/1
  Constant11/1 -> Data Store Write14/1
  Constant36/1 -> Data Store Write1/1
  Constant14/1 -> Data Store Write17/1
  Constant75/1 -> Data Store Write67/1
  Constant30/1 -> Data Store Write28/1
  Constant74/1 -> Data Store Write66/1
  Constant26/1 -> Divide5/2
  Constant15/1 -> Data Store Write18/1
  Divide4/1 -> Data Store Write24/1
  Constant10/1 -> Data Store Write13/1
  Constant21/1 -> Data Store Write36/1
  rpm_to_rad/s2/1 -> Divide1/1
  Constant44/1 -> Data Store Write38/1
  Constant28/1 -> Data Store Write23/1
  Divide3/1 -> Data Store Write10/1
  Constant1/1 -> Data Store Write2/1
  Constant32/1 -> Data Store Write32/1
  Constant9/1 -> Data Store Write12/1
  Constant7/1 -> Data Store Write8/1
  Constant25/1 -> Divide4/2
  Constant4/1 -> Data Store Write5/1
  rpm_to_rad/s4/1 -> Divide5/1
  Constant22/1 -> Data Store Write22/1
  Constant6/1 -> Data Store Write7/1
  Divide2/1 -> Data Store Write37/1
  Constant56/1 -> Data Store Write49/1
  Constant12/1 -> Data Store Write15/1
  rpm_to_rad/s1/1 -> Divide2/1
  Constant77/1 -> Data Store Write25/1
  Constant3/1 -> Data Store Write4/1
  Constant39/1 -> Data Store Write40/1
  Constant27/1 -> rpm_to_rad/s4/1
  Constant29/1 -> Data Store Write27/1
  Constant42/1 -> rpm_to_rad/s1/1
  Constant73/1 -> Data Store Write65/1
  Constant17/1 -> Data Store Write20/1
  Constant20/1 -> Data Store Write21/1
  Constant8/1 -> Data Store Write9/1
  Constant35/1 -> Data Store Write30/1, Data Store Write11/1
  Constant/1 -> Divide4/1
  Divide1/1 -> Data Store Write45/1
  Constant19/1 -> Divide3/2
  Constant38/1 -> Data Store Write39/1
  Constant23/1 -> Divide1/2
  Constant72/1 -> Data Store Write64/1
  Constant51/1 -> rpm_to_rad/s2/1
  Constant34/1 -> Data Store Write34/1

== system Target_Control_System/Target_Control_System/Simulation Controls/Simulation Data Store Initialization/setPositionControlModeTilt()/Enabled Subsystem ==
  note: // Valid for VP and tilt, use updateIqSetpointMax(blah) for prop though;
  Enable : EnablePort
  Constant : Constant  Value=0  OutDataTypeStr=uint32  SampleTime=-1
  Constant1 : Constant  Value=I_SET_MAX_INIT__TILT_TIP  OutDataTypeStr=single  SampleTime=-1
  Constant2 : Constant  Value=I_SET_MAX_INIT__TILT_LINKAGE  OutDataTypeStr=single  SampleTime=-1
  Constant3 : Constant  OutDataTypeStr=int32  SampleTime=-1
  Constant4 : Constant  OutDataTypeStr=uint32  SampleTime=-1
  Constant5 : Constant  Value=0  OutDataTypeStr=uint32  SampleTime=-1
  Constant6 : Constant  Value=0  OutDataTypeStr=uint32  SampleTime=-1
  Constant7 : Constant  Value=0  OutDataTypeStr=single  SampleTime=-1
  Constant8 : Constant  Value=0  OutDataTypeStr=single  SampleTime=-1
  Constant9 : Constant  Value=0  OutDataTypeStr=single  SampleTime=-1
  Data Store Read : DataStoreRead  DataStoreName=oTilt  DataStoreElements=oTilt.oMot_.oState_.oPosSensor_.iTiltReadheadCompensationEnabled_  IndexOptions=Index vector (dialog)  Indices=1  OutputSizes=1
  Data Store Read1 : DataStoreRead  Commented=on  DataStoreName=oTilt  DataStoreElements=oTilt.oMot_.oParam_.ePositionControlMode_  IndexOptions=Index vector (dialog)  Indices=1  OutputSizes=1
  Data Store Read{2..8} (7 alike) : DataStoreRead  DataStoreName=oTilt  DataStoreElements=oTilt.oMot_.oParam_.fIqSetpointMax_  IndexOptions=Index vector (dialog)  Indices=1  OutputSizes=1
  Data Store Write : DataStoreWrite  DataStoreName=oTilt  DataStoreElements=oTilt.oMot_.oParam_.uiTorqueMirroringActive_  IndexOptions=Index vector (dialog)  Indices=1  OutputSizes=1
  Data Store Write1 : DataStoreWrite  DataStoreName=oTilt  DataStoreElements=oTilt.oMot_.oParam_.fISetpointMax_  IndexOptions=Index vector (dialog)  Indices=1  OutputSizes=1
  Data Store Write10 : DataStoreWrite  DataStoreName=oTilt  DataStoreElements=oTilt.oMot_.oParam_.oPid2DataRpmCtrl_.oParameter_.fDMax_  IndexOptions=Index vector (dialog)  Indices=1  OutputSizes=1
  Data Store Write11 : DataStoreWrite  DataStoreName=oTilt  DataStoreElements=oTilt.oMot_.oParam_.oPid2DataRpmCtrl_.oParameter_.fOutMin_  IndexOptions=Index vector (dialog)  Indices=1  OutputSizes=1
  Data Store Write12 : DataStoreWrite  DataStoreName=oTilt  DataStoreElements=oTilt.oMot_.oParam_.oPid2DataRpmCtrl_.oParameter_.fOutMax_  IndexOptions=Index vector (dialog)  Indices=1  OutputSizes=1
  Data Store Write13 : DataStoreWrite  Commented=on  DataStoreName=oTilt  DataStoreElements=oTilt.oMot_.oParam_.ePositionControlMode_  IndexOptions=Index vector (dialog)  Indices=1  OutputSizes=1
  Data Store Write14 : DataStoreWrite  DataStoreName=oTilt  DataStoreElements=oTilt.oMot_.oParam_.oPid2DataRpmCtrl_.oParameter_.fIntegratorLeakFactor_  IndexOptions=Index vector (dialog)  Indices=1  OutputSizes=1
  Data Store Write15 : DataStoreWrite  DataStoreName=oTilt  DataStoreElements=oTilt.oMot_.oParam_.oPid2DataRpmCtrl_.oParameter_.fErrorReduction_  IndexOptions=Index vector (dialog)  Indices=1  OutputSizes=1
  Data Store Write16 : DataStoreWrite  DataStoreName=oTilt  DataStoreElements=oTilt.oMot_.oState_.oPosSensor_.oPidDataPosCtrl_.oParameter_.fErrorReduction_  IndexOptions=Index vector (dialog)  Indices=1  OutputSizes=1
  Data Store Write2 : DataStoreWrite  DataStoreName=oTilt  DataStoreElements=oTilt.oMot_.oState_.oPosSensor_.iPosControlEnabled_  IndexOptions=Index vector (dialog)  Indices=1  OutputSizes=1
  Data Store Write3 : DataStoreWrite  DataStoreName=oTilt  DataStoreElements=oTilt.oMot_.oState_.uiSpeedControllerActive_  IndexOptions=Index vector (dialog)  Indices=1  OutputSizes=1
  Data Store Write4 : DataStoreWrite  DataStoreName=oTilt  DataStoreElements=oTilt.oMot_.oOut_.uiForcedAngle_  IndexOptions=Index vector (dialog)  Indices=1  OutputSizes=1
  Data Store Write5 : DataStoreWrite  DataStoreName=oTilt  DataStoreElements=oTilt.oMot_.oParam_.iForcedPositionHoldMode_  IndexOptions=Index vector (dialog)  Indices=1  OutputSizes=1
  Data Store Write6 : DataStoreWrite  DataStoreName=oTilt  DataStoreElements=oTilt.oMot_.oParam_.fIqSetpointMax_  IndexOptions=Index vector (dialog)  Indices=1  OutputSizes=1
  Data Store Write7 : DataStoreWrite  DataStoreName=oTilt  DataStoreElements=oTilt.oMot_.oParam_.oPid2DataRpmCtrl_.oParameter_.fIntMin_  IndexOptions=Index vector (dialog)  Indices=1  OutputSizes=1
  Data Store Write8 : DataStoreWrite  DataStoreName=oTilt  DataStoreElements=oTilt.oMot_.oParam_.oPid2DataRpmCtrl_.oParameter_.fIntMax_  IndexOptions=Index vector (dialog)  Indices=1  OutputSizes=1
  Data Store Write9 : DataStoreWrite  DataStoreName=oTilt  DataStoreElements=oTilt.oMot_.oParam_.oPid2DataRpmCtrl_.oParameter_.fDMin_  IndexOptions=Index vector (dialog)  Indices=1  OutputSizes=1
  Enumerated Constant : simulink/Sources/Enumerated Constant  Commented=on  OutDataTypeStr=Enum: EPositionControlModes_t  Value=EPositionControlModes_t.ePassiveHolding  SampleTime=inf
  Switch : Switch  Criteria=u2 > Threshold
  Switch Case : SwitchCase  Commented=on  CaseConditions={EPositionControlModes_t.eNormal,EPositionControlModes_t.eNormalWithDeadZone,EPositionControlModes_t.eTorqueMirror,EPositionControlModes_t.ePassiveHolding}  ShowDefaultCase=off
  Switch Case Action Subsystem eNormal : Subsystem  Commented=on  TreatAsAtomicUnit=on
  Switch Case Action Subsystem eNormalWithDeadZone : Subsystem  Commented=on  TreatAsAtomicUnit=on
  Switch Case Action Subsystem ePassiveHolding : Subsystem  Commented=on  TreatAsAtomicUnit=on
  Switch Case Action Subsystem eTorqueMirror : Subsystem  Commented=on  TreatAsAtomicUnit=on
  Unary Minus : UnaryMinus
  Unary Minus1 : UnaryMinus
  Unary Minus2 : UnaryMinus
  wires:
  Constant7/1 -> Data Store Write14/1
  Constant8/1 -> Data Store Write15/1
  Constant9/1 -> Data Store Write16/1
  Unary Minus2/1 -> Data Store Write11/1
  Unary Minus/1 -> Data Store Write9/1
  Unary Minus1/1 -> Data Store Write7/1
  Constant/1 -> Data Store Write/1
  Data Store Read/1 -> Switch/2
  Switch/1 -> Data Store Write1/1
  Constant1/1 -> Switch/1
  Constant2/1 -> Switch/3
  Constant3/1 -> Data Store Write2/1
  Constant4/1 -> Data Store Write3/1
  Constant5/1 -> Data Store Write4/1
  Constant6/1 -> Data Store Write5/1
  Data Store Read1/1 -> Switch Case/1
  Switch Case/4 -> Switch Case Action Subsystem ePassiveHolding/Action
  Switch Case/3 -> Switch Case Action Subsystem eTorqueMirror/Action
  Switch Case/2 -> Switch Case Action Subsystem eNormalWithDeadZone/Action
  Switch Case/1 -> Switch Case Action Subsystem eNormal/Action
  Data Store Read2/1 -> Data Store Write6/1
  Data Store Read3/1 -> Unary Minus1/1
  Data Store Read4/1 -> Data Store Write8/1
  Data Store Read5/1 -> Unary Minus/1
  Data Store Read6/1 -> Data Store Write10/1
  Data Store Read7/1 -> Unary Minus2/1
  Data Store Read8/1 -> Data Store Write12/1

== system Target_Control_System/Target_Control_System/Simulation Controls/Simulation Data Store Initialization/setTiltMotorSpecificParameters()/Enabled Subsystem MotorType ==
  note: // Nacelles 1, 4-6 // The only difference between 1/4 and 5/6 is the range of motion. 1/4 go to 125 degrees nominally, 5/6 only to 110 degrees
  Enable : EnablePort
  Constant : Constant  SampleTime=-1
  Data Store Read : DataStoreRead  Commented=on  DataStoreName=oTilt  DataStoreElements=oTilt.oMot_.oParam_.fISetpointMax_  IndexOptions=Index vector (dialog)  Indices=1  OutputSizes=1
  Data Store Read1 : DataStoreRead  Commented=on  DataStoreName=oTilt  DataStoreElements=oTilt.oMot_.oState_.oPosSensor_.fGbxAngleMaxTrip_  IndexOptions=Index vector (dialog)  Indices=1  OutputSizes=1
  Data Store Read2 : DataStoreRead  Commented=on  DataStoreName=oTilt  DataStoreElements=oTilt.oMot_.oState_.oPosSensor_.fGbxAngleMinTrip_  IndexOptions=Index vector (dialog)  Indices=1  OutputSizes=1
  Data Store Write1 : DataStoreWrite  DataStoreName=oTilt  DataStoreElements=oTilt.oMot_.oParam_.oPid2DataRpmCtrl_.oParameter_.fOutMin_  IndexOptions=Index vector (dialog)  Indices=1  OutputSizes=1
  Data Store Write19 : DataStoreWrite  DataStoreName=oTilt  DataStoreElements=oTilt.oMot_.oParam_.oPid2DataRpmCtrl_.oParameter_.fOutMax_  IndexOptions=Index vector (dialog)  Indices=1  OutputSizes=1
  Data Store Write2 : DataStoreWrite  DataStoreName=oTilt  DataStoreElements=oTilt.oMot_.oParam_.oPid2DataRpmCtrl_.oParameter_.fIntMax_  IndexOptions=Index vector (dialog)  Indices=1  OutputSizes=1
  Data Store Write20 : DataStoreWrite  DataStoreName=oTilt  DataStoreElements=oTilt.oMot_.oState_.oPosSensor_.fActuatorSensorAngleMaxTrip_  IndexOptions=Index vector (dialog)  Indices=1  OutputSizes=1
  Data Store Write29 : DataStoreWrite  DataStoreName=oTilt  DataStoreElements=oTilt.oMot_.oState_.oPosSensor_.fGbxAngleMaxTrip_  IndexOptions=Index vector (dialog)  Indices=1  OutputSizes=1
  Data Store Write3 : DataStoreWrite  DataStoreName=oTilt  DataStoreElements=oTilt.oMot_.oParam_.oPid2DataRpmCtrl_.oParameter_.fIntMin_  IndexOptions=Index vector (dialog)  Indices=1  OutputSizes=1
  Data Store Write30 : DataStoreWrite  DataStoreName=oTilt  DataStoreElements=oTilt.oMot_.oState_.oPosSensor_.fGbxAngleMinTrip_  IndexOptions=Index vector (dialog)  Indices=1  OutputSizes=1
  Data Store Write4 : DataStoreWrite  DataStoreName=oTilt  DataStoreElements=oTilt.oMot_.oState_.oPosSensor_.fActuatorSensorAngleMinTrip_  IndexOptions=Index vector (dialog)  Indices=1  OutputSizes=1
  Data Store Write9 : DataStoreWrite  DataStoreName=oTilt  DataStoreElements=oTilt.oMot_.oParam_.fISetpointMax_  IndexOptions=Index vector (dialog)  Indices=1  OutputSizes=1
  Merge : Merge
  Merge1 : Merge
  Merge2 : Merge
  Switch Case : SwitchCase  CaseConditions={[1,2],3}  ShowDefaultCase=off
  Switch Case Action Subsystem MotorType12 : Subsystem  TreatAsAtomicUnit=on
  Switch Case Action Subsystem MotorType3 : Subsystem  TreatAsAtomicUnit=on
  wires:
  Switch Case/1 -> Switch Case Action Subsystem MotorType12/Action
  Switch Case/2 -> Switch Case Action Subsystem MotorType3/Action
  Constant/1 -> Switch Case/1
  Merge1/1 -> Data Store Write29/1, Data Store Write20/1
  Switch Case Action Subsystem MotorType3/2(maxTrip) -> Merge1/1
  Switch Case Action Subsystem MotorType12/2(maxTrip) -> Merge1/2
  Switch Case Action Subsystem MotorType3/1(IsetpointMax) -> Merge/2
  Switch Case Action Subsystem MotorType12/1(IsetpointMax) -> Merge/1
  Switch Case Action Subsystem MotorType12/3(minTrip) -> Merge2/2
  Switch Case Action Subsystem MotorType3/3(minTrip) -> Merge2/1
  Merge2/1 -> Data Store Write30/1, Data Store Write4/1
  Merge/1 -> Data Store Write9/1, Data Store Write3/1, Data Store Write2/1, Data Store Write1/1, Data Store Write19/1

== system Target_Control_System/Target_Control_System/Simulation Controls/Simulation Data Store Initialization/setupIirFilters(&oTilt)/computeCoefficientsButter() ==
  fCutoffFrequencyHz : Inport  OutDataTypeStr=single
  dSampleFrequencyHz : Inport  Port=2  OutDataTypeStr=single
  Add : Sum  Inputs=+++  OutDataTypeStr=double
  Add1 : Sum  Inputs=-+
  Add2 : Sum  Inputs=+-+  OutDataTypeStr=double
  Constant : Constant  Value=0.0008  OutDataTypeStr=single  SampleTime=-1
  Constant1 : Constant  Value=0.45  OutDataTypeStr=single  SampleTime=-1
  Constant{5,7,9..10} (4 alike) : Constant  SampleTime=-1
  Constant2 : Constant  Value=pi  OutDataTypeStr=double  SampleTime=-1
  Constant3 : Constant  OutDataTypeStr=double  SampleTime=-1
  Constant4 : Constant  Value=sqrt(2)  OutDataTypeStr=double  SampleTime=-1
  Constant6 : Constant  OutDataTypeStr=double  SampleTime=-1
  Constant8 : Constant  Value=2  SampleTime=-1
  Data Type Conversion : DataTypeConversion  OutDataTypeStr=double
  Divide : Product  Inputs=**  OutDataTypeStr=single
  Divide1 : Product  Inputs=**  OutDataTypeStr=single
  Divide{3,5..6,8,10..11} (6 alike) : Product  Inputs=**  OutDataTypeStr=double
  Divide2 : Product  Inputs=*/  OutDataTypeStr=double
  Divide4 : Product  Inputs=*/  OutDataTypeStr=double
  Divide7 : Product  Inputs=*/  OutDataTypeStr=double
  Divide9 : Product  Inputs=***  OutDataTypeStr=double
  Gain : Gain  Gain=2  OutDataTypeStr=double
  Gain1 : Gain  Gain=-1  OutDataTypeStr=double
  Gain2 : Gain  Gain=-1  OutDataTypeStr=double
  Gain3 : Gain  Gain=-1  OutDataTypeStr=double
  Mux : Mux  Inputs=6
  Saturation Dynamic : simulink/Discontinuities/Saturation Dynamic  OutMin=[]  OutMax=[]  OutDataTypeStr=Inherit: Same as second input  OutDataType=fixdt(1, 16)  OutScaling=2^-10  DoSatur=off
  Tan : Trigonometry  Operator=tan
  dpOutArray : Outport
  fCutoffFrequencyHz_out : Outport  Port=2
  wires:
  Saturation Dynamic/1 -> Data Type Conversion/1, fCutoffFrequencyHz_out/1  "fCutoffFrequencyHz"
  Data Type Conversion/1 -> Divide2/1
  Constant10/1 -> Mux/4
  [dA2] -> Gain3/1
  Gain3/1 -> Mux/6
  [dA1] -> Gain2/1
  Gain2/1 -> Mux/5
  [dB2] -> Mux/3
  [dB1] -> Mux/2
  [dB0] -> Mux/1
  Divide11/1 -> [dA2]
  Gain1/1 -> Divide11/2
  Add2/1 -> Gain1/1
  Constant9/1 -> Add2/3
  Divide10/1 -> Add2/2
  [kdQ] -> Divide10/2
  Constant7/1 -> Add1/1
  Divide8/1 -> Add1/2, Add2/1
  Divide9/1 -> [dA1]
  Constant8/1 -> Divide9/3
  Add1/1 -> Divide9/2
  [kdIta] -> Divide8/1, Divide8/2, Divide10/1
  Gain/1 -> [dB1]
  Divide7/1 -> [dB0], Gain/1, [dB2], Divide9/1, Divide11/1
  Add/1 -> Divide7/2
  Constant6/1 -> Divide7/1
  Constant5/1 -> Add/3
  Divide5/1 -> Add/2
  Divide6/1 -> Add/1
  [kdQ] -> Divide5/2
  [kdIta] -> Divide5/1, Divide6/1, Divide6/2
  Mux/1 -> dpOutArray/1
  Constant4/1 -> [kdQ]
  Divide4/1 -> [kdIta]
  Constant3/1 -> Divide4/1
  Tan/1 -> Divide4/2
  Divide3/1 -> Tan/1
  Constant2/1 -> Divide3/2
  Divide2/1 -> Divide3/1  "dFf"
  Constant/1 -> Divide/2
  fCutoffFrequencyHz/1 -> Saturation Dynamic/2  "fCutoffFrequencyHz"
  Divide1/1 -> Saturation Dynamic/1
  dSampleFrequencyHz/1 -> Divide1/2, Divide2/2, Divide/1
  Constant1/1 -> Divide1/1
  Divide/1 -> Saturation Dynamic/3
